simulink model "motorSimPWM"  (R2019b)
settings: Solver=VariableStepAuto  StartTime=0.0  StopTime=10.0  RelTol=1e-3
values from neighbouring files (symbols this model uses):
  b = 0.5    [MotorExpScriptIdent.m]    (also in motorSimScript.m; motorSimScriptIdent.m)
  J = 0.05    [MotorExpScriptIdent.m]    (also in motorSimScript.m; motorSimScriptIdent.m)
  Ke = 0.5    [MotorExpScriptIdent.m]    (also in motorSimScript.m; motorSimScriptIdent.m)
  Kt = 0.5    [MotorExpScriptIdent.m]    (also in motorSimScript.m; motorSimScriptIdent.m)
  Ra = 1    [MotorExpScriptIdent.m]    (also in motorSimScript.m; motorSimScriptIdent.m)
libraries: simulink x2
settings Model: Creator=coffe  LastModifiedBy=coffe

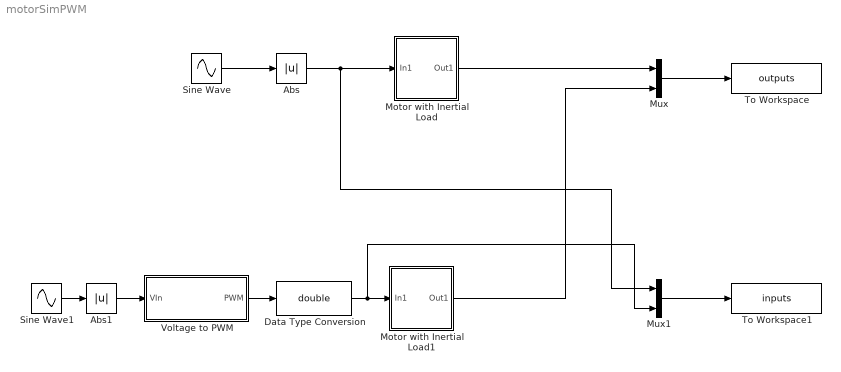
== system motorSimPWM ==
  Abs : Abs
  Abs1 : Abs
  Data Type Conversion : DataTypeConversion  OutDataTypeStr=double
  Motor with Inertial Load : Subsystem
  Motor with Inertial Load1 : Subsystem
  Mux : Mux  Inputs=2
  Mux1 : Mux  Inputs=2
  Sine Wave : Sin  SampleTime=0
  Sine Wave1 : Sin  SampleTime=0
  To Workspace : ToWorkspace  VariableName=outputs  SaveFormat=Timeseries  SampleTime=-1
  To Workspace1 : ToWorkspace  VariableName=inputs  SaveFormat=Timeseries  SampleTime=-1
  Voltage to PWM : Subsystem
  wires:
  Sine Wave/1 -> Abs/1
  Abs/1 -> Mux1/1, Motor with Inertial Load/1(In1)
  Motor with Inertial Load/1(Out1) -> Mux/1
  Voltage to PWM/1(PWM) -> Data Type Conversion/1
  Mux/1 -> To Workspace/1
  Sine Wave1/1 -> Abs1/1
  Motor with Inertial Load1/1(Out1) -> Mux/2
  Abs1/1 -> Voltage to PWM/1(VIn)
  Data Type Conversion/1 -> Mux1/2, Motor with Inertial Load1/1(In1)
  Mux1/1 -> To Workspace1/1

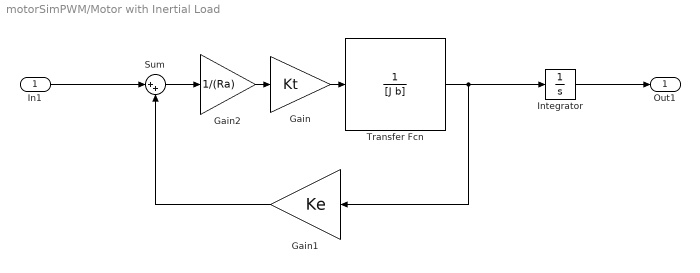
== system motorSimPWM/Motor with Inertial Load ==
  In1 : Inport
  Gain : Gain  Gain=Kt
  Gain1 : Gain  Gain=Ke
  Gain2 : Gain  Gain=1/(Ra)
  Integrator : Integrator
  Sum : Sum  Inputs=|++
  Transfer Fcn : TransferFcn  Denominator=[J b]
  Out1 : Outport
  wires:
  Gain/1 -> Transfer Fcn/1
  Transfer Fcn/1 -> Integrator/1, Gain1/1
  Gain2/1 -> Gain/1
  In1/1 -> Sum/1
  Gain1/1 -> Sum/2
  Sum/1 -> Gain2/1
  Integrator/1 -> Out1/1

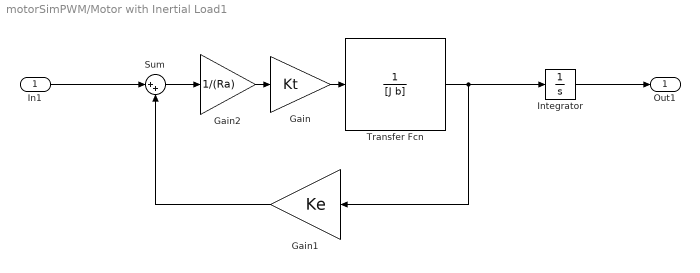
== system motorSimPWM/Motor with Inertial Load1 ==
  In1 : Inport
  Gain : Gain  Gain=Kt
  Gain1 : Gain  Gain=Ke
  Gain2 : Gain  Gain=1/(Ra)
  Integrator : Integrator
  Sum : Sum  Inputs=|++
  Transfer Fcn : TransferFcn  Denominator=[J b]
  Out1 : Outport
  wires:
  Gain/1 -> Transfer Fcn/1
  Transfer Fcn/1 -> Integrator/1, Gain1/1
  Gain2/1 -> Gain/1
  In1/1 -> Sum/1
  Gain1/1 -> Sum/2
  Sum/1 -> Gain2/1
  Integrator/1 -> Out1/1

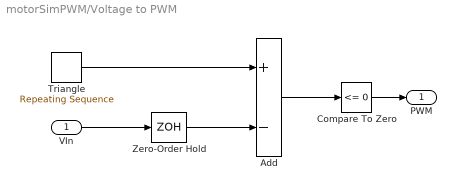
== system motorSimPWM/Voltage to PWM ==
  VIn : Inport
  Add : Sum  Inputs=+-  SampleTime=1/10000
  Compare To Zero : simulink/Logic and Bit Operations/Compare To Zero  relop=<=  OutDataTypeStr=uint8
  Triangle : simulink/Sources/Repeating Sequence  rep_seq_t=[0 1/100/4 3/100/4 1/100]*25  rep_seq_y=[0.5 0 1 0.5]
  Zero-Order Hold : ZeroOrderHold  SampleTime=1/10000
  PWM : Outport  VectorParamsAs1DForOutWhenUnconnected=off
  wires:
  Triangle/1 -> Add/1
  VIn/1 -> Zero-Order Hold/1
  Add/1 -> Compare To Zero/1
  Compare To Zero/1 -> PWM/1
  Zero-Order Hold/1 -> Add/2
